simulink model "RC"  (Simulink 7.1)
settings: Solver=ode45  StartTime=0.0  StopTime=.001  RelTol=1e-3
undefined symbols (not defined in the file): C, R, V
settings Model: Creator=Smrit  LastModifiedBy=Smrit

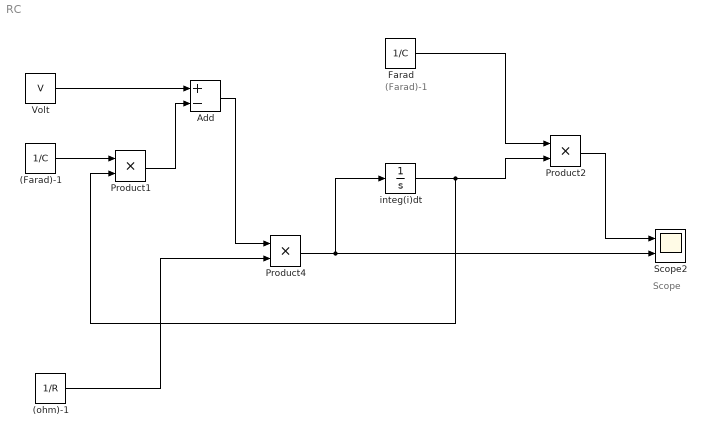
== system RC ==
  note: Scope
  note: (Farad)-1
  (Farad)-1 : Constant  Value=1/C  OutDataType=sfix(16)  OutScaling=2^0
  (ohm)-1 : Constant  Value=1/R  OutDataType=sfix(16)  OutScaling=2^0
  Add : Sum  Inputs=+-  OutDataType=sfix(16)  OutScaling=2^-10
  Farad : Constant  Value=1/C  OutDataType=sfix(16)  OutScaling=2^0
  Product1 : Product  OutDataType=sfix(16)  OutScaling=2^0  RndMeth=Zero
  Product2 : Product  OutDataType=sfix(16)  OutScaling=2^0  RndMeth=Zero
  Product4 : Product  OutDataType=sfix(16)  OutScaling=2^0  RndMeth=Zero
  Scope2 : Scope  NumInputPorts=2
      settings: YMin=-5~-5  YMax=5~5
  Volt : Constant  Value=V  OutDataType=sfix(16)  OutScaling=2^0
  integ(i)dt : Integrator
  wires:
  integ(i)dt/1 -> Product2/2, Product1/2
  (ohm)-1/1 -> Product4/2
  Product4/1 -> Scope2/2, integ(i)dt/1
  Farad/1 -> Product2/1
  Product2/1 -> Scope2/1
  Volt/1 -> Add/1
  Product1/1 -> Add/2
  Add/1 -> Product4/1
  (Farad)-1/1 -> Product1/1
